simulink model "section_2"  (R2024b)
settings: Solver=VariableStepAuto  StartTime=0.0  StopTime=10.0  RelTol=1e-3
settings Model: Creator=amand  LastModifiedBy=amand

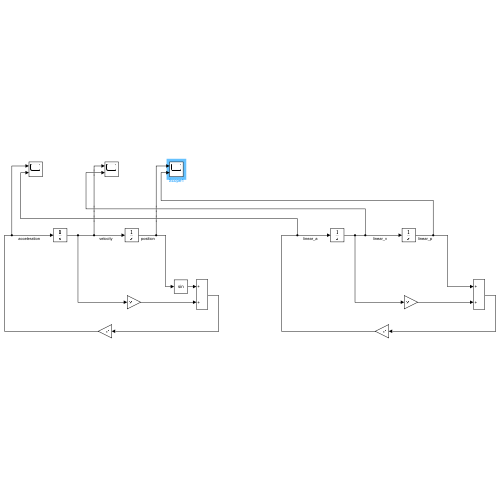
[thumbnail: Simulink's stored preview of the top-level diagram]
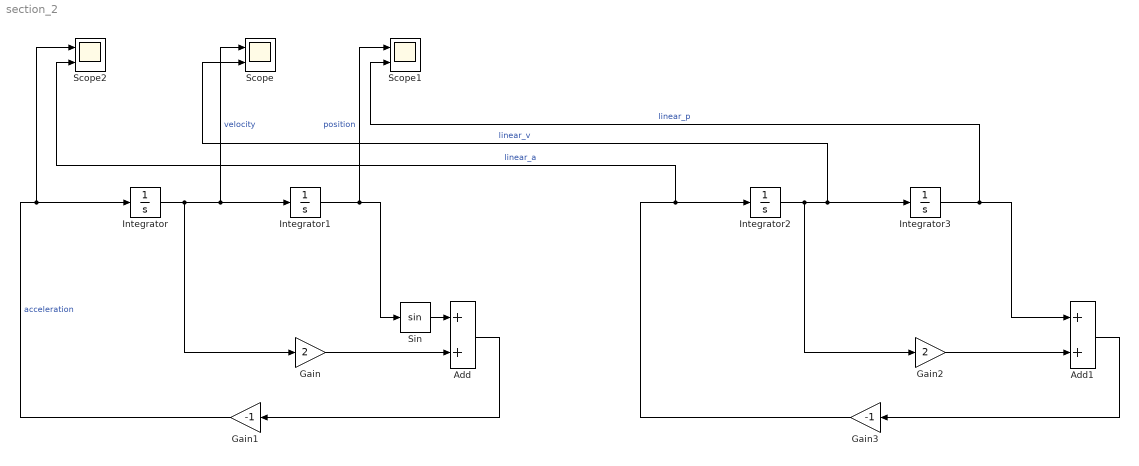
== system section_2 ==
  Add : Sum
  Add1 : Sum
  Gain : Gain  Gain=2
  Gain1 : Gain  Gain=-1
  Gain2 : Gain  Gain=2
  Gain3 : Gain  Gain=-1
  Integrator : Integrator  InitialCondition=1
  Integrator1 : Integrator  InitialCondition=2
  Integrator2 : Integrator  InitialCondition=1
  Integrator3 : Integrator  InitialCondition=2
  Scope : Scope  NumInputPorts=2
  Scope1 : Scope  NumInputPorts=2
  Scope2 : Scope  NumInputPorts=2
  Sin : Trigonometry
  wires:
  Integrator/1 -> Gain/1, Scope/1, Integrator1/1  "velocity"
  Integrator1/1 -> Scope1/1, Sin/1  "position"
  Add/1 -> Gain1/1
  Gain/1 -> Add/2
  Sin/1 -> Add/1
  Gain1/1 -> Scope2/1, Integrator/1  "acceleration"
  Add1/1 -> Gain3/1
  Gain3/1 -> Scope2/2, Integrator2/1  "linear_a"
  Integrator3/1 -> Scope1/2, Add1/1  "linear_p"
  Gain2/1 -> Add1/2
  Integrator2/1 -> Gain2/1, Scope/2, Integrator3/1  "linear_v"
